simulink model "StreamingLS"  (R2018b)
settings: Solver=FixedStepAuto  StartTime=1  StopTime=10  FixedStep=1  RelTol=1e-3
libraries: hdlsllib x5, simulink x1
settings Model: Creator=jason  LastModifiedBy=jason
settings OptimizationCC: DefaultParameterBehavior=Inlined
settings DebuggingCC: ParameterOverflowMsg=warning

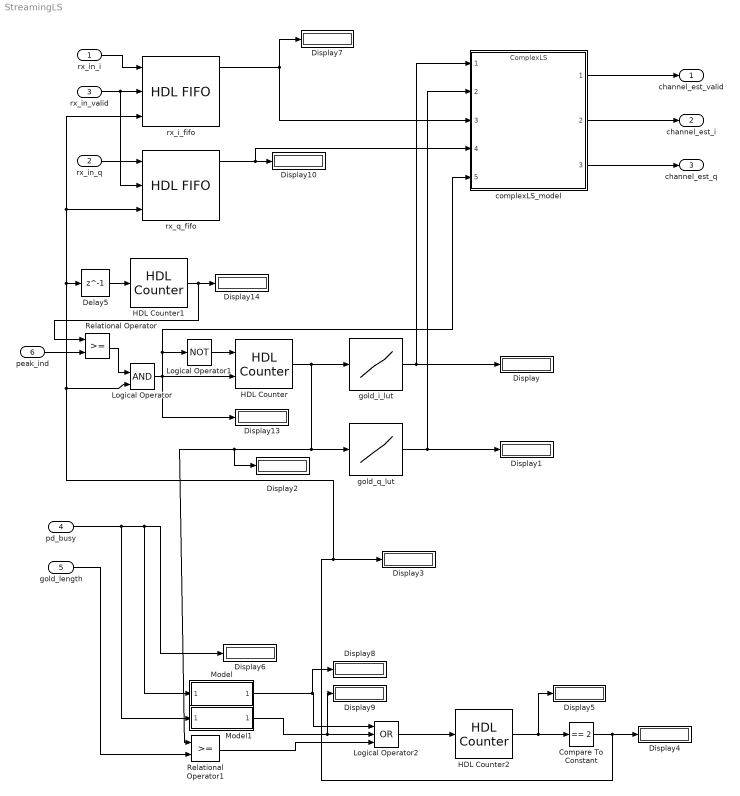
== system StreamingLS ==
  rx_in_i : Inport  OutDataTypeStr=fixdt(1,16,15)  SampleTime=1  Interpolate=off
  rx_in_q : Inport  Port=2  OutDataTypeStr=fixdt(1,16,15)  SampleTime=1  Interpolate=off
  rx_in_valid : Inport  Port=3  OutDataTypeStr=boolean  SampleTime=1  Interpolate=off
  pd_busy : Inport  Port=4  OutDataTypeStr=boolean  SampleTime=1  Interpolate=off
  gold_length : Inport  Port=5  OutDataTypeStr=uint16  SampleTime=1  Interpolate=off
  peak_ind : Inport  Port=6  OutDataTypeStr=uint16  SampleTime=1  Interpolate=off
  Compare To Constant : simulink/Logic and Bit Operations/Compare To Constant  relop===  const=2  OutDataTypeStr=boolean
  Delay5 : Delay  DelayLength=1
  Display{,1..10,13..14} (13 alike) : Display
      Display13 settings: Format=decimal (Stored Integer)
      Display14 settings: Format=decimal (Stored Integer)
      Display2 settings: Format=decimal (Stored Integer)
  HDL Counter : hdlsllib/Sources/HDL Counter  CountType=Free running  CountInit=1  CountStep=1  CountMax=25  CountFromType=Initial value  CountFrom=1  CountResetPort=on  CountLoadPort=off  CountEnbPort=on  CountDirPort=off  CountDataType=Unsigned  CountWordLen=16  CountFracLen=0  CountSampTime=1
      settings: SourceProductBaseCode=HD
  HDL Counter1 : hdlsllib/Sources/HDL Counter  CountType=Free running  CountInit=1  CountStep=1  CountMax=25  CountFromType=Initial value  CountFrom=1  CountResetPort=off  CountLoadPort=off  CountEnbPort=on  CountDirPort=off  CountDataType=Unsigned  CountWordLen=16  CountFracLen=0  CountSampTime=1
      settings: SourceProductBaseCode=HD
  HDL Counter2 : hdlsllib/Sources/HDL Counter  CountType=Count limited  CountInit=0  CountStep=1  CountMax=2  CountFromType=Initial value  CountFrom=0  CountResetPort=off  CountLoadPort=off  CountEnbPort=on  CountDirPort=off  CountDataType=Unsigned  CountWordLen=16  CountFracLen=0  CountSampTime=1
      settings: SourceProductBaseCode=HD
  Logical Operator : Logic  IconShape=distinctive  AllPortsSameDT=off  OutDataTypeStr=boolean
  Logical Operator1 : Logic  Operator=NOT  IconShape=distinctive  AllPortsSameDT=off  OutDataTypeStr=boolean
  Logical Operator2 : Logic  Operator=OR  Inputs=3  IconShape=distinctive  AllPortsSameDT=off  OutDataTypeStr=boolean
  Model : ModelReference  ModelNameDialog=re_detect  SimulationMode=Normal  ModelReferenceVersion=1.6
  Model1 : ModelReference  ModelNameDialog=fe_detect  SimulationMode=Normal  ModelReferenceVersion=1.3
  Relational Operator : RelationalOperator  OutDataTypeStr=boolean  RndMeth=Nearest
  Relational Operator1 : RelationalOperator  OutDataTypeStr=boolean  RndMeth=Nearest
  complexLS_model : ModelReference  ModelNameDialog=ComplexLS.slx  SimulationMode=Normal  ModelReferenceVersion=1.172
  gold_i_lut : Lookup_n-D  NumberOfTableDimensions=1  LookupTableObject=''  BreakpointsForDimension1=uint16([1:100]);  BreakpointsForDimension1FirstPoint=10  BreakpointsForDimension2FirstPoint=10  BreakpointsForDimension1Spacing=12  BreakpointsForDimension2Spacing=12  IndexSearchMethod=Evenly spaced points  Table=[0.1538; 0.2282; 0.2753; 0.2904; 0.2678; 0.2226; 0.1475; 0.0555; -0.0424; -0.1347; -0.2101; -0.2594; -0.2722; -0.2594; -0.2101; -0.1347; -0.0424; 0.0555; 0.1475; 0.2226; 0.2763; 0.2977; 0.2794; 0.2276; 0.1477; 0.0478; -0.0623; -0.1725; -0.2689; -0.3564; -0.4163; -0.4493; -0.4546; -0.4329; -0.3872; -0.3214; -0.2364; -0.1508; -0.0581; 0.0313; 0.1114; 0.1768; 0.2233; 0.2478; 0.2445; 0.2267; 0.1835; 0.1230; 0.0499; -0.0298; -0.1101; -0.1852; -0.2545; -0.3086; -0.3404; -0.3536; -0.3500; -0.3325; -0.3055; -0.2736; -0.2459; -0.2136; -0.1926; -0.1807; -0.1788; -0.1865; -0.2027; -0.2254; -0.2478; -0.2799; -0.3056; -0.3262; -0.3387; -0.3401; -0.3282; -0.3015; -0.2637; -0.2106; -0.1396; -0.0592; 0.0251; 0.1067; 0.1795; 0.2379; 0.2826; 0.3069; 0.3069; 0.2909; 0.2651; 0.2369; 0.2138; 0.2018; 0.2005; 0.2156; 0.2494; 0.2914; 0.3326; 0.3631; 0.3737; 0.3572]'  TableDataTypeStr=fixdt(1,16,15)  InterpMethod=Flat  InternalRulePriority=Speed  OutDataTypeStr=fixdt(1,16,15)  RndMeth=Simplest  InputSameDT=on
  gold_q_lut : Lookup_n-D  NumberOfTableDimensions=1  LookupTableObject=''  BreakpointsForDimension1=uint16([1:100]);  BreakpointsForDimension1FirstPoint=10  BreakpointsForDimension2FirstPoint=10  BreakpointsForDimension1Spacing=12  BreakpointsForDimension2Spacing=12  IndexSearchMethod=Evenly spaced points  Table=[0.1538; 0.2282; 0.2753; 0.2904; 0.2678; 0.2226; 0.1475; 0.0555; -0.0424; -0.1347; -0.2101; -0.2594; -0.2722; -0.2594; -0.2101; -0.1347; -0.0424; 0.0555; 0.1475; 0.2226; 0.2763; 0.2977; 0.2794; 0.2276; 0.1477; 0.0478; -0.0623; -0.1725; -0.2689; -0.3564; -0.4163; -0.4493; -0.4546; -0.4329; -0.3872; -0.3214; -0.2364; -0.1508; -0.0581; 0.0313; 0.1114; 0.1768; 0.2233; 0.2478; 0.2445; 0.2267; 0.1835; 0.1230; 0.0499; -0.0298; -0.1101; -0.1852; -0.2545; -0.3086; -0.3404; -0.3536; -0.3500; -0.3325; -0.3055; -0.2736; -0.2459; -0.2136; -0.1926; -0.1807; -0.1788; -0.1865; -0.2027; -0.2254; -0.2478; -0.2799; -0.3056; -0.3262; -0.3387; -0.3401; -0.3282; -0.3015; -0.2637; -0.2106; -0.1396; -0.0592; 0.0251; 0.1067; 0.1795; 0.2379; 0.2826; 0.3069; 0.3069; 0.2909; 0.2651; 0.2369; 0.2138; 0.2018; 0.2005; 0.2156; 0.2494; 0.2914; 0.3326; 0.3631; 0.3737; 0.3572]'  TableDataTypeStr=fixdt(1,16,15)  InterpMethod=Flat  InternalRulePriority=Speed  OutDataTypeStr=fixdt(1,16,15)  RndMeth=Simplest  InputSameDT=on
  rx_i_fifo : hdlsllib/HDL RAMs/HDL FIFO  fifo_size=1024  ratio=1  push_msg=Warning  pop_msg=Warning  show_empty=on  show_full=on  show_num=on
      settings: SourceProductName=HDL Coder  SourceProductBaseCode=HD
  rx_q_fifo : hdlsllib/HDL RAMs/HDL FIFO  fifo_size=1024  ratio=1  push_msg=Warning  pop_msg=Warning  show_empty=on  show_full=on  show_num=on
      settings: SourceProductName=HDL Coder  SourceProductBaseCode=HD
  channel_est_valid : Outport  OutDataTypeStr=boolean
  channel_est_i : Outport  Port=2  OutDataTypeStr=fixdt(1,16,14)
  channel_est_q : Outport  Port=3  OutDataTypeStr=fixdt(1,16,14)
  wires:
  rx_in_i/1 -> rx_i_fifo/1
  rx_in_valid/1 -> rx_q_fifo/2, rx_i_fifo/2
  rx_in_q/1 -> rx_q_fifo/1
  gold_q_lut/1 -> complexLS_model/2, Display1/1
  gold_i_lut/1 -> complexLS_model/1, Display/1
  HDL Counter/1 -> gold_i_lut/1, gold_q_lut/1, Relational Operator1/1, Display2/1
  pd_busy/1 -> Model1/1, Model/1, Display6/1
  gold_length/1 -> Relational Operator1/2
  rx_i_fifo/1 -> complexLS_model/3, Display7/1
  rx_q_fifo/1 -> complexLS_model/4, Display10/1
  Delay5/1 -> HDL Counter1/1
  HDL Counter1/1 -> Display14/1, Relational Operator/1
  peak_ind/1 -> Relational Operator/2
  Logical Operator/1 -> Display13/1, Logical Operator1/1, complexLS_model/5, HDL Counter/2
  Relational Operator/1 -> Logical Operator/1
  Compare To Constant/1 -> Delay5/1, rx_q_fifo/3, rx_i_fifo/3, Logical Operator/2, Display3/1, Display4/1
  complexLS_model/1 -> channel_est_valid/1
  complexLS_model/3 -> channel_est_q/1
  complexLS_model/2 -> channel_est_i/1
  Logical Operator1/1 -> HDL Counter/1
  Model/1 -> Display8/1, Logical Operator2/1
  Model1/1 -> Display9/1, Logical Operator2/2
  Relational Operator1/1 -> Logical Operator2/3
  HDL Counter2/1 -> Display5/1, Compare To Constant/1
  Logical Operator2/1 -> HDL Counter2/1
